simulink model "r_controller_system_integrated"  (R2025b)
settings: Solver=ode45  StartTime=0.0  StopTime=0.25  FixedStep=1e-05  MaxStep=1e-06  RelTol=1e-3
values from neighbouring files (symbols this model uses):
  params = Simulink.Parameter(params_data)    [r_controller_calc_params.m]    (also in r_controller_calc_params_p2.m)
undefined symbols (not defined in the file or in its folder): Amplitude, Channel, d, Frequency, Phase, SignalType, StepTime
libraries: simulink x3
settings Model: Creator=PME406_01  LastModifiedBy=PME406_01
settings DebuggingCC: MergeDetectMultiDrivingBlocksExec=none
settings ModelReferenceCC: PropagateSignalLabelsOutOfModel=off

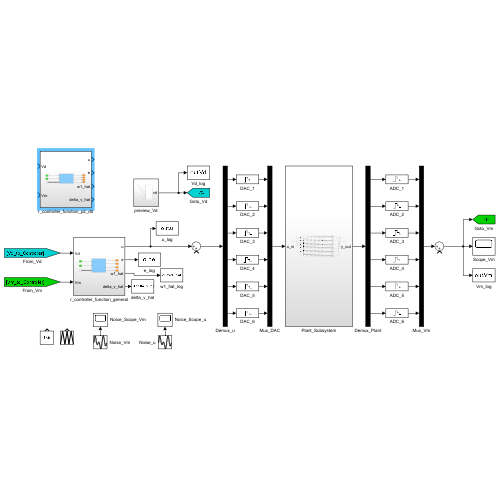
[thumbnail: Simulink's stored preview of the top-level diagram]
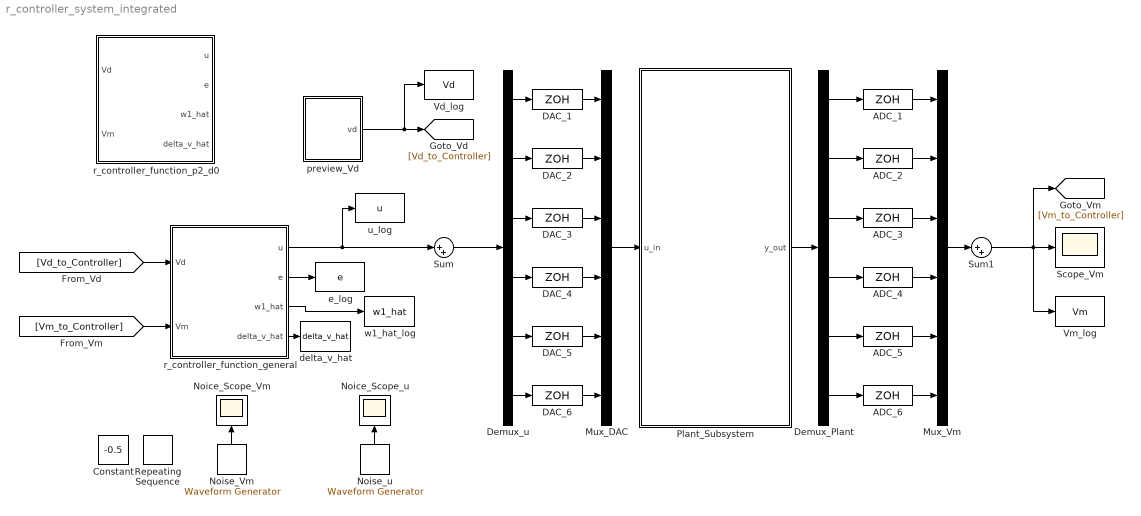
== system r_controller_system_integrated ==
  ADC_{1..6} (6 alike) : ZeroOrderHold  SampleTime=1e-05
  Constant : Constant  Value=-0.5
  DAC_{1..6} (6 alike) : ZeroOrderHold  SampleTime=1e-05
  Demux_Plant : Demux  Outputs=6
  Demux_u : Demux  Outputs=6
  Mux_DAC : Mux  Inputs=6
  Mux_Vm : Mux  Inputs=6
  Noice_Scope_Vm : Scope
      settings: DataLoggingSaveFormat=Array
  Noice_Scope_u : Scope
      settings: DataLoggingSaveFormat=Array
  Noise_Vm : simulink/Sources/Waveform Generator  OutMin=[]  OutMax=[]  OutDataTypeStr=double  SelectedSignal=4  Signals=sin(0.01,50*2*pi, 0) + sin(0.01, 1000*2*pi, pi/2) +sin(0.01,500*2*pi, pi/4)#square(0.01,1000*2*pi,0,50)+square(0.01,500*2*pi,pi/2,50)+square(0.01,50*2*pi,pi/4,50)#sin(0.02,100*2*pi, pi/4)+sin(0.02,3200*2*pi, 0)#square(0.005,10*2*pi,0,50)##sawtooth(0.02,50*2*pi, 0) + sawtooth(0.02, 1000*2*pi, pi/2) +sawtooth(0.02,500*2*pi, pi/4)  BlockNames=MultiportSwitch_75be51d97721476#MultiportSwitch_30160a8004a3476#MultiportSwitch_4637dbd864f54f8#MultiportSwitch_6fc3281f74a1493#MultiportSwitch_6d08dda3201040f#MultiportSwitch_d71c5f632a8a412  SampleTime=1e-5
  Noise_u : simulink/Sources/Waveform Generator  OutMin=[]  OutMax=[]  OutDataTypeStr=double  SelectedSignal=4  Signals=sin(0.1,50*2*pi, 0) + sin(0.1, 1000*2*pi, pi/2) +sin(0.1,500*2*pi, pi/4)#square(0.1,1000*2*pi,0,50)+square(0.1,500*2*pi,0,50)+square(0.1,50*2*pi,0,50)#sin(0.1,100*2*pi, pi/4)+sin(0.1,3000*2*pi,0)#square(0.1,1000*2*pi,pi/4,50)##sawtooth(0.1,50*2*pi, 0) + sawtooth(0.1, 1000*2*pi, pi/2) +sawtooth(0.1,500*2*pi, pi/4)  BlockNames=MultiportSwitch_0ff2f2b35e8d4a7#MultiportSwitch_4c68b0874292414#MultiportSwitch_7d8d7ea2149c456#MultiportSwitch_121c1283fd924f3#MultiportSwitch_5c21996da7fd48f#MultiportSwitch_cbcb2585dc95419  SampleTime=1e-5
  Plant_Subsystem : Subsystem
  Repeating Sequence : simulink/Sources/Repeating Sequence  rep_seq_t=[0 0.0005 0.001]  rep_seq_y=[-0.02 0.02 -0.02]
  Scope_Vm : Scope
      settings: DataLoggingSaveFormat=Array
  Sum : Sum  Inputs=|++
  Sum1 : Sum  Inputs=|++
  Vd_log : ToWorkspace  VariableName=Vd  SampleTime=1e-5
      settings: Save2DSignal=2-D array (concatenate along first dimension)
  Vm_log : ToWorkspace  VariableName=Vm  SampleTime=1e-5
      settings: Save2DSignal=2-D array (concatenate along first dimension)
  delta_v_hat : ToWorkspace  VariableName=delta_v_hat  SampleTime=1e-5
      settings: Save2DSignal=2-D array (concatenate along first dimension)
  e_log : ToWorkspace  VariableName=e  SampleTime=1e-5
      settings: Save2DSignal=2-D array (concatenate along first dimension)
  preview_Vd : Subsystem
  r_controller_function_general : Subsystem
  r_controller_function_p2_d0 : Subsystem
  u_log : ToWorkspace  VariableName=u  SampleTime=1e-5
      settings: Save2DSignal=2-D array (concatenate along first dimension)
  w1_hat_log : ToWorkspace  VariableName=w1_hat  SampleTime=1e-5
      settings: Save2DSignal=2-D array (concatenate along first dimension)
  wires:
  ADC_6/1 -> Mux_Vm/6
  Demux_u/5 -> DAC_5/1
  DAC_4/1 -> Mux_DAC/4
  ADC_2/1 -> Mux_Vm/2
  Demux_u/6 -> DAC_6/1
  ADC_4/1 -> Mux_Vm/4
  DAC_3/1 -> Mux_DAC/3
  DAC_1/1 -> Mux_DAC/1
  DAC_2/1 -> Mux_DAC/2
  Demux_u/1 -> DAC_1/1
  Plant_Subsystem/1(y_out) -> Demux_Plant/1
  Demux_Plant/2 -> ADC_2/1
  Demux_Plant/5 -> ADC_5/1
  ADC_3/1 -> Mux_Vm/3
  ADC_1/1 -> Mux_Vm/1
  Demux_Plant/4 -> ADC_4/1
  DAC_5/1 -> Mux_DAC/5
  Demux_u/3 -> DAC_3/1
  Demux_Plant/3 -> ADC_3/1
  Demux_Plant/1 -> ADC_1/1
  DAC_6/1 -> Mux_DAC/6
  Demux_u/4 -> DAC_4/1
  Mux_DAC/1 -> Plant_Subsystem/1(u_in)
  Demux_u/2 -> DAC_2/1
  ADC_5/1 -> Mux_Vm/5
  Demux_Plant/6 -> ADC_6/1
  preview_Vd/1(vd) -> Vd_log/1, [Vd_to_Controller]
  Sum/1 -> Demux_u/1
  Noise_Vm/1 -> Noice_Scope_Vm/1
  Mux_Vm/1 -> Sum1/1
  Sum1/1 -> Vm_log/1, [Vm_to_Controller], Scope_Vm/1
  Noise_u/1 -> Noice_Scope_u/1
  r_controller_function_general/4(delta_v_hat) -> delta_v_hat/1
  [Vd_to_Controller] -> r_controller_function_general/1(Vd)
  [Vm_to_Controller] -> r_controller_function_general/2(Vm)
  r_controller_function_general/3(w1_hat) -> w1_hat_log/1
  r_controller_function_general/2(e) -> e_log/1
  r_controller_function_general/1(u) -> u_log/1, Sum/1

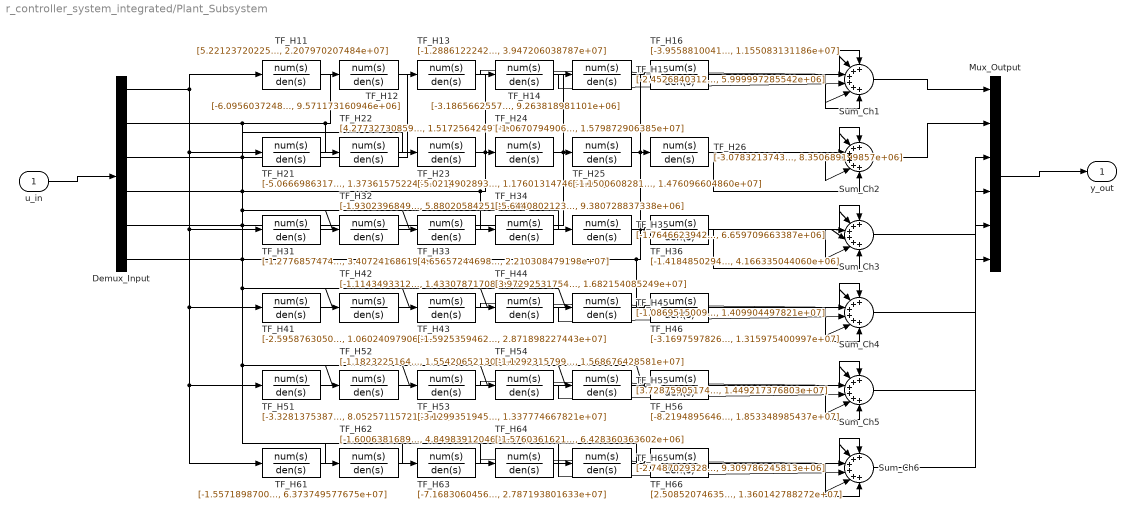
== system r_controller_system_integrated/Plant_Subsystem ==
  u_in : Inport
  Demux_Input : Demux  Outputs=6
  Mux_Output : Mux  Inputs=6
  Sum_Ch{1..6} (6 alike) : Sum  Inputs=++++++
  TF_H11 : TransferFcn  Numerator=[5.221237202258e+06]  Denominator=[1, 1.125476429798e+04, 2.207970207484e+07]
  TF_H12 : TransferFcn  Numerator=[-6.095603724823e+04]  Denominator=[1, 1.615096196557e+03, 9.571173160946e+06]
  TF_H13 : TransferFcn  Numerator=[-1.288612224236e+06]  Denominator=[1, 1.231137597589e+04, 3.947206038787e+07]
  TF_H14 : TransferFcn  Numerator=[-3.186566255776e+05]  Denominator=[1, 7.765927137710e+03, 9.263818981101e+06]
  TF_H15 : TransferFcn  Numerator=[-2.452684031253e+05]  Denominator=[1, 5.746401647961e+03, 5.999997285542e+06]
  TF_H16 : TransferFcn  Numerator=[-3.955881004140e+05]  Denominator=[1, 3.580306515557e+03, 1.155083131186e+07]
  TF_H21 : TransferFcn  Numerator=[-5.066698631790e+04]  Denominator=[1, 1.108261849372e+03, 1.373615752245e+07]
  TF_H22 : TransferFcn  Numerator=[4.277327308593e+06]  Denominator=[1, 1.003268373777e+04, 1.517256424974e+07]
  TF_H23 : TransferFcn  Numerator=[-5.021490289304e+05]  Denominator=[1, 8.810895080316e+03, 1.176013147465e+07]
  TF_H24 : TransferFcn  Numerator=[-1.067079490600e+06]  Denominator=[1, 1.135112820448e+04, 1.579872906385e+07]
  TF_H25 : TransferFcn  Numerator=[-1.150060828107e+06]  Denominator=[1, 1.065992916636e+04, 1.476096604860e+07]
  TF_H26 : TransferFcn  Numerator=[-3.078321374306e+05]  Denominator=[1, 6.847783968129e+03, 8.350689199857e+06]
  TF_H31 : TransferFcn  Numerator=[-1.277685747428e+06]  Denominator=[1, 1.368269686933e+04, 3.407241686199e+07]
  TF_H32 : TransferFcn  Numerator=[-1.930239684968e+05]  Denominator=[1, 4.560870597302e+03, 5.880205842512e+06]
  TF_H33 : TransferFcn  Numerator=[4.656572446985e+06]  Denominator=[1, 9.513164457161e+03, 2.210308479198e+07]
  TF_H34 : TransferFcn  Numerator=[-5.644080212304e+04]  Denominator=[1, 1.954878812118e+03, 9.380728837338e+06]
  TF_H35 : TransferFcn  Numerator=[-1.764662394212e+05]  Denominator=[1, 5.122349981324e+03, 6.659709663387e+06]
  TF_H36 : TransferFcn  Numerator=[-1.418485029440e+05]  Denominator=[1, 1.438504147902e+03, 4.166335044060e+06]
  TF_H41 : TransferFcn  Numerator=[-2.595876305066e+05]  Denominator=[1, 7.070165651413e+03, 1.060240979066e+07]
  TF_H42 : TransferFcn  Numerator=[-1.114349331223e+06]  Denominator=[1, 9.846928206402e+03, 1.433078717084e+07]
  TF_H43 : TransferFcn  Numerator=[-1.592535946272e+05]  Denominator=[1, 2.790294019501e+03, 2.871898227443e+07]
  TF_H44 : TransferFcn  Numerator=[3.972925317547e+06]  Denominator=[1, 1.159715140811e+04, 1.682154085249e+07]
  TF_H45 : TransferFcn  Numerator=[-1.086951500933e+06]  Denominator=[1, 1.075231371220e+04, 1.409904497821e+07]
  TF_H46 : TransferFcn  Numerator=[-3.169759782656e+05]  Denominator=[1, 8.067558736035e+03, 1.315975400997e+07]
  TF_H51 : TransferFcn  Numerator=[-3.328137538766e+05]  Denominator=[1, 7.227274813518e+03, 8.052571157216e+06]
  TF_H52 : TransferFcn  Numerator=[-1.182322516481e+06]  Denominator=[1, 1.030784744910e+04, 1.554206521303e+07]
  TF_H53 : TransferFcn  Numerator=[-3.129935194599e+05]  Denominator=[1, 7.870328655037e+03, 1.337774667821e+07]
  TF_H54 : TransferFcn  Numerator=[-1.129231579925e+06]  Denominator=[1, 1.104821595243e+04, 1.568676428581e+07]
  TF_H55 : TransferFcn  Numerator=[3.728759051745e+06]  Denominator=[1, 1.050075182774e+04, 1.449217376803e+07]
  TF_H56 : TransferFcn  Numerator=[-8.219489564647e+04]  Denominator=[1, 1.407969854523e+03, 1.853348985437e+07]
  TF_H61 : TransferFcn  Numerator=[-1.557189870041e+06]  Denominator=[1, 2.234640585923e+04, 6.373749577675e+07]
  TF_H62 : TransferFcn  Numerator=[-1.600638168987e+05]  Denominator=[1, 3.864055922471e+03, 4.849839120469e+06]
  TF_H63 : TransferFcn  Numerator=[-7.168306045699e+05]  Denominator=[1, 9.251556589809e+03, 2.787193801633e+07]
  TF_H64 : TransferFcn  Numerator=[-1.576036162155e+05]  Denominator=[1, 4.743270970318e+03, 6.428360363602e+06]
  TF_H65 : TransferFcn  Numerator=[-2.748702932822e+04]  Denominator=[1, 4.876033357949e+02, 9.309786245813e+06]
  TF_H66 : TransferFcn  Numerator=[2.508520746356e+06]  Denominator=[1, 5.985310903650e+03, 1.360142788272e+07]
  y_out : Outport
  wires:
  Sum_Ch3/1 -> Mux_Output/3
  TF_H36/1 -> Sum_Ch3/6
  TF_H16/1 -> Sum_Ch1/6
  TF_H63/1 -> Sum_Ch6/3
  Demux_Input/2 -> TF_H52/1, TF_H62/1, TF_H42/1, TF_H32/1, TF_H12/1, TF_H22/1
  TF_H23/1 -> Sum_Ch2/3
  TF_H31/1 -> Sum_Ch3/1
  Sum_Ch1/1 -> Mux_Output/1
  TF_H51/1 -> Sum_Ch5/1
  TF_H12/1 -> Sum_Ch1/2
  TF_H61/1 -> Sum_Ch6/1
  TF_H22/1 -> Sum_Ch2/2
  Demux_Input/4 -> TF_H54/1, TF_H64/1, TF_H44/1, TF_H14/1, TF_H24/1, TF_H34/1
  TF_H14/1 -> Sum_Ch1/4
  TF_H62/1 -> Sum_Ch6/2
  TF_H25/1 -> Sum_Ch2/5
  Sum_Ch4/1 -> Mux_Output/4
  TF_H41/1 -> Sum_Ch4/1
  TF_H45/1 -> Sum_Ch4/5
  Sum_Ch6/1 -> Mux_Output/6
  TF_H54/1 -> Sum_Ch5/4
  TF_H64/1 -> Sum_Ch6/4
  TF_H55/1 -> Sum_Ch5/5
  Demux_Input/6 -> TF_H56/1, TF_H66/1, TF_H16/1, TF_H26/1, TF_H36/1, TF_H46/1
  TF_H42/1 -> Sum_Ch4/2
  TF_H13/1 -> Sum_Ch1/3
  TF_H26/1 -> Sum_Ch2/6
  TF_H21/1 -> Sum_Ch2/1
  Demux_Input/5 -> TF_H55/1, TF_H65/1, TF_H45/1, TF_H15/1, TF_H25/1, TF_H35/1
  Sum_Ch2/1 -> Mux_Output/2
  u_in/1 -> Demux_Input/1
  TF_H44/1 -> Sum_Ch4/4
  TF_H24/1 -> Sum_Ch2/4
  TF_H66/1 -> Sum_Ch6/6
  TF_H43/1 -> Sum_Ch4/3
  TF_H33/1 -> Sum_Ch3/3
  TF_H52/1 -> Sum_Ch5/2
  Demux_Input/3 -> TF_H53/1, TF_H63/1, TF_H43/1, TF_H33/1, TF_H13/1, TF_H23/1
  TF_H15/1 -> Sum_Ch1/5
  TF_H56/1 -> Sum_Ch5/6
  TF_H32/1 -> Sum_Ch3/2
  TF_H34/1 -> Sum_Ch3/4
  TF_H53/1 -> Sum_Ch5/3
  Demux_Input/1 -> TF_H51/1, TF_H61/1, TF_H41/1, TF_H31/1, TF_H21/1, TF_H11/1
  TF_H11/1 -> Sum_Ch1/1
  TF_H35/1 -> Sum_Ch3/5
  Mux_Output/1 -> y_out/1
  Sum_Ch5/1 -> Mux_Output/5
  TF_H65/1 -> Sum_Ch6/5
  TF_H46/1 -> Sum_Ch4/6

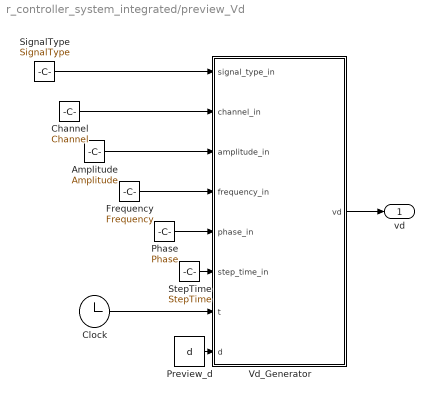
== system r_controller_system_integrated/preview_Vd ==
  Amplitude : Constant  Value=Amplitude
  Channel : Constant  Value=Channel
  Clock : Clock
  Frequency : Constant  Value=Frequency
  Phase : Constant  Value=Phase
  Preview_d : Constant  Value=d
  SignalType : Constant  Value=SignalType
  StepTime : Constant  Value=StepTime
  Vd_Generator : MATLAB Function  TreatAsAtomicUnit=on
  vd : Outport
  wires:
  Clock/1 -> Vd_Generator/7(t)
  Frequency/1 -> Vd_Generator/4(frequency_in)
  SignalType/1 -> Vd_Generator/1(signal_type_in)
  StepTime/1 -> Vd_Generator/6(step_time_in)
  Phase/1 -> Vd_Generator/5(phase_in)
  Amplitude/1 -> Vd_Generator/3(amplitude_in)
  Channel/1 -> Vd_Generator/2(channel_in)
  Vd_Generator/1(vd) -> vd/1
  Preview_d/1 -> Vd_Generator/8(d)

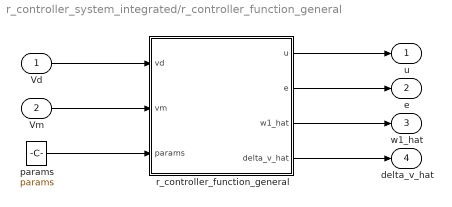
== system r_controller_system_integrated/r_controller_function_general ==
  Vd : Inport
  Vm : Inport  Port=2
  params : Constant  Value=params  OutDataTypeStr=Bus: ParamsBus
  r_controller_function_general : MATLAB Function  TreatAsAtomicUnit=on
  u : Outport
  e : Outport  Port=2
  w1_hat : Outport  Port=3
  delta_v_hat : Outport  Port=4
  wires:
  r_controller_function_general/3(w1_hat) -> w1_hat/1
  r_controller_function_general/2(e) -> e/1
  Vm/1 -> r_controller_function_general/2(vm)
  Vd/1 -> r_controller_function_general/1(vd)
  r_controller_function_general/1(u) -> u/1
  params/1 -> r_controller_function_general/3(params)
  r_controller_function_general/4(delta_v_hat) -> delta_v_hat/1

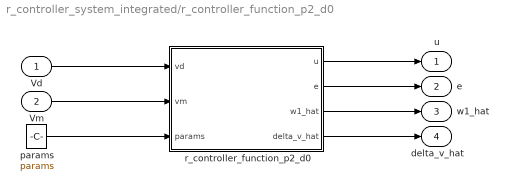
== system r_controller_system_integrated/r_controller_function_p2_d0 ==
  Vd : Inport
  Vm : Inport  Port=2
  params : Constant  Value=params  OutDataTypeStr=Bus: ParamsBus
  r_controller_function_p2_d0 : MATLAB Function  TreatAsAtomicUnit=on
  u : Outport
  e : Outport  Port=2
  w1_hat : Outport  Port=3
  delta_v_hat : Outport  Port=4
  wires:
  Vm/1 -> r_controller_function_p2_d0/2(vm)
  Vd/1 -> r_controller_function_p2_d0/1(vd)
  r_controller_function_p2_d0/1(u) -> u/1
  r_controller_function_p2_d0/2(e) -> e/1
  r_controller_function_p2_d0/3(w1_hat) -> w1_hat/1
  params/1 -> r_controller_function_p2_d0/3(params)
  r_controller_function_p2_d0/4(delta_v_hat) -> delta_v_hat/1

== matlab function r_controller_system_integrated/r_controller_function_general/r_controller_function_general ==
  settings: updateMethod=DISCRETE  sampleTime=1e-5
  data: vd input size=6; u output size=6; vm input size=6; e output size=6; w1_hat output size=6; params input; delta_v_hat output size=6
function [u, e, w1_hat, delta_v_hat] = r_controller_function_general(vd, vm, params)
    % R Controller with Pre-calculated Parameters
    %
    % Implements R Controller using pre-calculated parameters from
    % r_controller_calc_params(). This function contains ONLY the
    % difference equations for real-time execution.
    %
    % Inputs:
    %   vd     - Desired voltage [6×1] (may be preview vd[k+d])
    %   vm     - Measured voltage [6×1]
    %   params - Controller parameters (structure from r_controller_calc_params)
    %
    % Outputs:
    %   u      - Control input [6×1]
    %   e      - Tracking error [6×1] (δv = vf - vm)
    %   w1_hat - Disturbance estimate [6×1]
    %   delta_v_hat - Estimated tracking error [6×1] (δv̂)
    %
    % Variable naming convention:
    %   - Addition: A (e.g., one_A_beta = 1 + beta)
    %   - Subtraction: S (e.g., one_S_bc = 1 - bc)
    %   - Multiplication: M (e.g., b_M_lambda_c = b * lambda_c)
    %   - Negative: neg_ (e.g., neg_beta = -beta)

    % ====================================================================
    % PERSISTENT STATE VARIABLES
    % ====================================================================
    persistent vd_k1 vd_k2           % vd[k-1], vd[k-2] - Input history
    persistent vf_k1 vf_k2           % vf[k-1], vf[k-2] - Filtered vd history
    persistent delta_v_k1            % δv[k-1] - Tracking error history
    persistent delta_v_hat_k1        % δv̂[k-1] - Estimated error history
    persistent w1_hat_k1 w2_hat_k1   % ŵ1[k-1], ŵ2[k-1] - Disturbance estimates
    persistent delta_vc_k1 delta_vc_k2  % δvc[k-1], δvc[k-2] - Compensated error history
    persistent uc_k1 uc_k2           % uc[k-1], uc[k-2] - Control output history
    persistent initialized

    % ====================================================================
    % INITIALIZATION
    % ====================================================================
    if isempty(initialized)
        initialized = true;
        vd_k1 = zeros(6, 1);
        vd_k2 = zeros(6, 1);
        vf_k1 = zeros(6, 1);
        vf_k2 = zeros(6, 1);
        delta_v_k1 = zeros(6, 1);
        delta_v_hat_k1 = zeros(6, 1);
        w1_hat_k1 = zeros(6, 1);
        w2_hat_k1 = zeros(6, 1);
        delta_vc_k1 = zeros(6, 1);
        delta_vc_k2 = zeros(6, 1);
        uc_k1 = zeros(6, 1);
        uc_k2 = zeros(6, 1);
    end

    % ====================================================================
    % FEEDFORWARD FILTER (vf calculation)
    % vf[k] = alpha_vf * {c0·vd[k] + c1·vd[k-1] + c2·vd[k-2]}
    % ====================================================================
    vf_k = params.alpha_vf * (params.c0_b * vd + ...
                               params.c1_one_S_b_M_lambda_c * vd_k1 + ...
                               params.c2_neg_lambda_c * vd_k2);

    % δvf[k] = vf[k] - (1-bc)·vf[k-1] - bc·vf[k-2]
    delta_vf = vf_k - params.one_S_bc * vf_k1 - params.bc * vf_k2;

    % δv[k] = vf[k] - vm[k]
    delta_v = vf_k - vm;

    % ====================================================================
    % ESTIMATOR (disturbance observer)
    % ====================================================================
    error_term = delta_v_k1 - delta_v_hat_k1;

    % δv̂[k] = λc·δv̂[k-1] + δvf[k] + L1·{δv[k-1] - δv̂[k-1]}
    delta_v_hat = params.lambda_c * delta_v_hat_k1 + delta_vf + params.L1 * error_term;

    % ŵ1[k] = (1+β)·ŵ1[k-1] - β·ŵ2[k-1] + L2·{δv[k-1] - δv̂[k-1]}
    w1_hat = params.one_A_beta * w1_hat_k1 + params.neg_beta * w2_hat_k1 + params.L2 * error_term;

    % ŵ2[k] = ŵ1[k-1] + L3·{δv[k-1] - δv̂[k-1]}
    w2_hat = w1_hat_k1 + params.L3 * error_term;

    % ====================================================================
    % CONTROL LAW
    % ====================================================================
    % δvc[k] = δv[k] - ŵ1[k]
    delta_vc = delta_v - w1_hat;

    % uc[k] = (1-bc)·uc[k-1] + bc·uc[k-2] + ku·{δvc[k] - a1·δvc[k-1] - a2·δvc[k-2]}
    uc = params.one_S_bc * uc_k1 + params.bc * uc_k2 + ...
         params.ku * (delta_vc - params.a1 * delta_vc_k1 - params.a2 * delta_vc_k2);

    % u[k] = B^-1 · uc[k]
    u = params.B_inv * uc;

    % e[k] = δv[k]
    e = delta_v;

    % ====================================================================
    % STATE UPDATES
    % ====================================================================
    vd_k2 = vd_k1;
    vd_k1 = vd;
    vf_k2 = vf_k1;
    vf_k1 = vf_k;
    delta_v_k1 = delta_v;
    delta_v_hat_k1 = delta_v_hat;
    w1_hat_k1 = w1_hat;
    w2_hat_k1 = w2_hat;
    delta_vc_k2 = delta_vc_k1;
    delta_vc_k1 = delta_vc;
    uc_k2 = uc_k1;
    uc_k1 = uc;
end

== matlab function r_controller_system_integrated/preview_Vd/Vd_Generator ==
  settings: updateMethod=DISCRETE  sampleTime=1e-5
  data: signal_type_in input; channel_in input; amplitude_in input; frequency_in input; phase_in input; step_time_in input; t input; vd output size=6; d input
function vd = fcn(signal_type_in, channel_in, amplitude_in, frequency_in, phase_in, step_time_in, t, d)

    Ts = 1e-5;  

    t_future = t + Ts * d;%<<<<<<<<<<<<<<<

    vd = zeros(6, 1);

    channel = round(channel_in);
    if channel < 1 || channel > 6
        channel = 1;
    end

    if signal_type_in == 1
        % Sine Wave
        vd(channel) = amplitude_in * sin(2*pi*frequency_in*t_future + 180 * phase_in /  pi);
    else
        if t_future >= step_time_in
            vd(channel) = amplitude_in;
        else
            vd(channel) = 0;
        end
    end
end

== matlab function r_controller_system_integrated/r_controller_function_p2_d0/r_controller_function_p2_d0 ==
  settings: updateMethod=DISCRETE  sampleTime=1e-5
  data: vd input size=6; u output size=6; vm input size=6; params input; e output; w1_hat output; delta_v_hat output size=6
function [u, e, w1_hat, delta_v_hat] = r_controller_function_p2_d0(vd, vm, params)
    % R Controller with d=0 (no preview) - Parameterized Version
    % Based on Page 2 equations but adapted for d=0
    %
    % Implements R Controller using pre-calculated parameters.
    % This version uses the Page 2 estimator gains (l_1 to l_4)
    % but with d=0 (no preview buffer).
    %
    % Inputs:
    %   vd     - Desired voltage [6×1]
    %   vm     - Measured voltage [6×1]
    %   params - Controller parameters (structure from r_controller_calc_params_p2)
    %
    % Outputs:
    %   u      - Control input [6×1]
    %   e      - Tracking error [6×1] (δv = vf - vm)
    %   w1_hat - Disturbance estimate [6×1]
    %   delta_v_hat - Estimated tracking error [6×1] (δv̂)

    % ====================================================================
    % PERSISTENT STATE VARIABLES
    % ====================================================================
    persistent vf vf_k1              % vf[k], vf[k-1] - Filtered vd
    persistent delta_vf_k1            % δvf[k-1]
    persistent delta_v_k1             % δv[k-1]
    persistent delta_v_hat_k1        % δv̂[k-1]
    persistent w1_hat_k1              % ŵ1[k-1]
    persistent delta_w_hat_k1         % δŵ[k-1]
    persistent w2_hat_k1              % ŵ2[k-1]
    persistent uc_k1 uc_k2            % uc[k-1], uc[k-2]
    persistent delta_vc_k1 delta_vc_k2  % δvc[k-1], δvc[k-2]
    persistent initialized

    % ====================================================================
    % INITIALIZATION
    % ====================================================================
    if isempty(initialized)
        initialized = true;
        vf = zeros(6, 1);
        vf_k1 = zeros(6, 1);
        delta_vf_k1 = zeros(6, 1);
        delta_v_k1 = zeros(6, 1);
        delta_v_hat_k1 = zeros(6, 1);
        w1_hat_k1 = zeros(6, 1);
        delta_w_hat_k1 = zeros(6, 1);
        w2_hat_k1 = zeros(6, 1);
        uc_k1 = zeros(6, 1);
        uc_k2 = zeros(6, 1);
        delta_vc_k1 = zeros(6, 1);
        delta_vc_k2 = zeros(6, 1);
    end

    % ====================================================================
    % FEEDFORWARD FILTER (d=0 version)
    % ====================================================================
    % For d=0, we need proper feedforward filter with kc
    % vf[k+1] = vd[k] (but scaled appropriately)
    vf_next = vd;

    % δvf[k] = vf[k+1] - (1-bc)·vf[k] - bc·vf[k-1]
    delta_vf = vf_next - params.one_S_bc * vf - params.bc * vf_k1;

    % δv[k] = vf[k] - vm[k]
    delta_v = vf - vm;

    % ====================================================================
    % ESTIMATOR (using Page 2 gains l_1, l_2, l_3, l_4)
    % ====================================================================
    error_term = delta_v_k1 - delta_v_hat_k1;

    % δv̂[k] = λc·δv̂[k-1] + δvf[k-1] + ℓ1·{δv[k-1] - δv̂[k-1]}
    delta_v_hat = params.lambda_c * delta_v_hat_k1 + delta_vf_k1 + params.l_1 * error_term;

    % ŵ1[k] = ŵ1[k-1] + δŵ[k-1] + ℓ2·{δv[k-1] - δv̂[k-1]}
    w1_hat = w1_hat_k1 + delta_w_hat_k1 + params.l_2 * error_term;

    % δŵ[k] = δŵ[k-1] + ℓ3·{δv[k-1] - δv̂[k-1]}
    delta_w_hat = delta_w_hat_k1 + params.l_3 * error_term;

    % ŵ2[k] = ŵ1[k-1] + ℓ4·{δv[k-1] - δv̂[k-1]}
    w2_hat = w1_hat_k1 + params.l_4 * error_term;

    % ====================================================================
    % CONTROL LAW
    % ====================================================================
    % δvc[k] = δv[k] - ŵ1[k]
    delta_vc = delta_v - w1_hat;

    % uc[k] = (1-bc)·uc[k-1] - bc·uc[k-2] + ku·{δvc[k] - a1·δvc[k-1] - a2·δvc[k-2]}
    % Note: The second term is negative bc (not positive as in general version)
    uc = params.one_S_bc * uc_k1 - params.bc * uc_k2 + ...
         params.ku * (delta_vc - params.a1 * delta_vc_k1 - params.a2 * delta_vc_k2);

    % u[k] = B^-1 · uc[k]
    u = params.B_inv * uc;

    % e[k] = δv[k]
    e = delta_v;

    % ====================================================================
    % STATE UPDATES
    % ====================================================================
    vf_k1 = vf;            % vf[k-1] ← vf[k]
    vf = vf_next;          % vf[k] ← vf[k+1]

    delta_vf_k1 = delta_vf;       % δvf[k-1] ← δvf[k]
    delta_v_k1 = delta_v;         % δv[k-1] ← δv[k]
    delta_v_hat_k1 = delta_v_hat; % δv̂[k-1] ← δv̂[k]
    w1_hat_k1 = w1_hat;           % ŵ1[k-1] ← ŵ1[k]
    delta_w_hat_k1 = delta_w_hat; % δŵ[k-1] ← δŵ[k]
    w2_hat_k1 = w2_hat;           % ŵ2[k-1] ← ŵ2[k]

    uc_k2 = uc_k1;                % uc[k-2] ← uc[k-1]
    uc_k1 = uc;                   % uc[k-1] ← uc[k]
    delta_vc_k2 = delta_vc_k1;    % δvc[k-2] ← δvc[k-1]
    delta_vc_k1 = delta_vc;       % δvc[k-1] ← δvc[k]
end
